simulink library "INT_CoESS_Dem"  (R2016b)
settings: Solver=VariableStepAuto  StartTime=0.0  StopTime=10.0  RelTol=1e-3
settings Model: Creator=Administrator  LastModifiedBy=Administrator

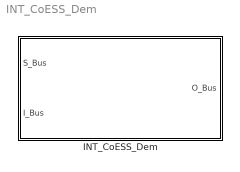
== system INT_CoESS_Dem ==
  INT_CoESS_Dem : Subsystem

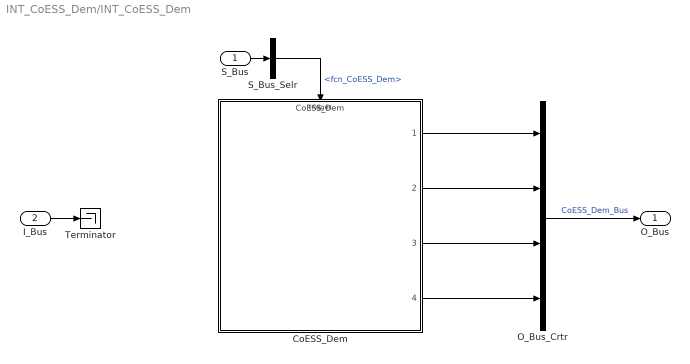
== system INT_CoESS_Dem/INT_CoESS_Dem ==
  S_Bus : Inport
  I_Bus : Inport  Port=2
  CoESS_Dem : ModelReference  ModelNameDialog=CoESS_Dem  SimulationMode=Normal  ModelReferenceVersion=1.3  TriggerPortName=function  TriggerPortTriggerType=function-call  TriggerPortStatesWhenEnabling=held
  O_Bus_Crtr : BusCreator  Inputs=4
  S_Bus_Selr : BusSelector  OutputSignals=fcn_CoESS_Dem
  Terminator : Terminator
  O_Bus : Outport
  wires:
  S_Bus_Selr/1 -> CoESS_Dem/Trigger  "<fcn_CoESS_Dem>"
  S_Bus/1 -> S_Bus_Selr/1
  I_Bus/1 -> Terminator/1
  O_Bus_Crtr/1 -> O_Bus/1  "CoESS_Dem_Bus"
  CoESS_Dem/1 -> O_Bus_Crtr/1
  CoESS_Dem/2 -> O_Bus_Crtr/2
  CoESS_Dem/3 -> O_Bus_Crtr/3
  CoESS_Dem/4 -> O_Bus_Crtr/4
